simulink model "FIR_Compiler_Ex2"  (R2023a)
settings: Solver=VariableStepAuto  StartTime=0.0  StopTime=1e4  RelTol=1e-3
undefined symbols (not defined in the file): c, S, vsva2197, xcvc1902
libraries: hdlBasic x7, hdlUtilities x4, aieUtilities x4, dspsrcs4 x3, dspmlti4 x1, hdlDSPIP x1, vmcUtilities x1
settings Model: Creator=abehbood  LastModifiedBy=robg

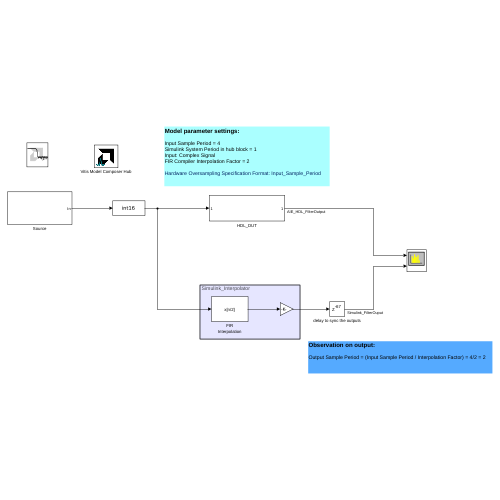
[thumbnail: Simulink's stored preview of the top-level diagram]
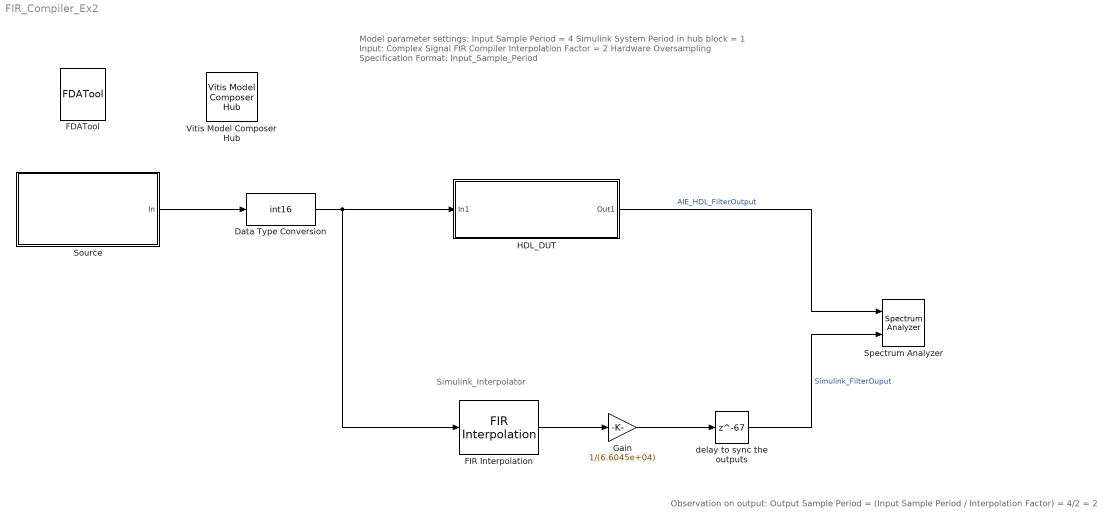
== system FIR_Compiler_Ex2 ==
  note: Simulink_Interpolator
  note: Model parameter settings:
      |
      | Input Sample Period = 4
      | Simulink System Period in hub block = 1
      | Input: Complex Signal
      | FIR Compiler Interpolation Factor = 2
      |
      | Hardware Oversampling Specification Format: Input_Sample_Period
  note: Observation on output:
      |
      | Output Sample Period = (Input Sample Period / Interpolation Factor) = 4/2 = 2
  Data Type Conversion : DataTypeConversion  OutDataTypeStr=int16  SaturateOnIntegerOverflow=off  RndMeth=Floor
  FDATool : hdlUtilities/FDATool  block_type=fdatool
      settings: infoedit=FDATool
  FIR Interpolation : dspmlti4/FIR Interpolation  FilterSource=Dialog parameters  PrivateCoeffs=0  h=[0,0,0,0,0,0,0,0,0,0,0,0,0,0,1,-1,1,-1,1,-1,1,-2,2,-2,3,-3,4,-4,5,-5,6,-7,8,-9,10,-11,12,-13,15,-17,18,-20,23,-25,27,-30,33,-36,40,-44,48,-52,56,-61,67,-72,78,-85,92,-99,107,-115,124,-134,144,-155,167,-179,192,-207,222,-238,256,-274,295,-316,340,-366,394,-424,458,-495,536,-581,633,-692,759,-837,929,-1040,1175,-1344,1564,-1862,2290,-2958,4156,-6944,20858,20858,-6944,4156,-2958,2290,-1862,1564,-1344,1175,-1040,929,-837,759,-692,633,-581,536,-495,458,-424,394,-366,340,-316,295,-274,256,-238,222,-207,192,-179,167,-155,144,-134,124,-115,107,-99,92,-85,78,-72,67,-61,56,-52,48,-44,40,-36,33,-30,27,-25,23,-20,18,-17,15,-13,12,-11,10,-9,8,-7,6,-5,5,-4,4,-3,3,-2,2,-2,1,-1,1,-1,1,-1,1,0,0,0,0,0,0,0,0,0,0,0,0,0,0]  L=2  FilterObject=FINTERP  framing=Enforce single-rate processing  outputBufInitCond=0  roundingMode=Floor  overflowMode=off  firstCoeffMode=Binary point scaling  firstCoeffWordLength=16  firstCoeffFracLength=0  firstCoeffDataTypeStr=fixdt(1,16,0)  firstCoeffMin=[]  firstCoeffMax=[]  firstCoeffLastDataTypeStr=fixdt(1,16,0)  outputDataTypeStr=Inherit: Same as accumulator  outputMin=[]  outputMax=[]  outputLastDataTypeStr=Inherit: Same as accumulator
  Gain : Gain  Gain=1/(6.6045e+04)  OutDataTypeStr=int16
  HDL_DUT : Subsystem
  Source : Subsystem
  Spectrum Analyzer : SpectrumAnalyzer  NumInputPorts=2  AveragingMethod=Exponential  ShowLegend=on  ChannelNames="[\"\"]"  DefaultConfigurationName=spbscopes.SpectrumAnalyzerBlockCfg
  Vitis Model Composer Hub : vmcUtilities/Vitis Model Composer Hub  Tag=genX  CodeGeneration=off  SubsystemName=filter_chain_DUT  StartColumn=1  NumberOfColumns=1  TargetDirectory=./code_hw_emu  exportDesign=off  analyzeDesign=off  validateDesignOnHw=off  ExportType=HW Code  IpVendor=xilinx.com  IpLibrary=hls  IpVersion=1.0  IpHWLanguage=Verilog  AieCompilerOptions={}  AieSimulatorOptions={}  CreateTestbench=off  TestbenchStackSize=10  RunRtlSim=off  RunCSim=off  RunAieSim=on  AieSimTimeout=50000  RunAieSimProfiling=off  LaunchVitisAnalyzer=off  PlotOutput=off  RunX86Sim=off  X86SimTimeout=10  GenHwImage=off  GenLibadfXo=off  GenHwValidationCode=off  PlatformType=Specify Platform  Platform=/proj/xbuilds/SWIP/2024.1_0306_2227/installs/lin64/Vitis/2024.1/base_platforms/xilinx_vck190_base_202410_1/xilinx_vck190_base_202410_1.xpfm  HwSystemType=Baremetal  HwValidationTarget=hw_emu  ProjDevice=Versal VCK190 Evaluation Platform (xcvc1902-vsva2197-2MP-e-S)  ProjDevicePart=xcvc1902-vsva2197-2MP-e-S  AIEType=AIE  SamplePeriod=-1  ClockFrequency=200  DataPathParallelism=1  xilinxfamily=versalaicore  part=xcvc1902  speed=-2MP-e-S  package=vsva2197  directory=./code_hw_emu/ip/PL/src  testbench=on  incr_netlist=off  synthesis_tool=Vivado  clock_wrapper=Clock Enables  dbl_ovrd=According to Block Masks  dcm_input_clock_period=10  sysclk_period=5  simulink_period=2  eval_field=0  IPInfoJsonString="{\"HDLSubsystem\":{\"SubsystemName\":\"PL\",\"IPName\":\"Subsystem\",\"IPLibrary\":\"VMC\",\"IPVendor\":\"User Company\",\"IPVersion\":\"1.0\",\"TargetDirectory\":\"./code_hw_emu\",\"SubsystemDir\":\"./code_hw_emu/ip/PL\"},\"SubsystemTag\":\"DUTNode\",\"AIESubsystem\":{\"SubsystemName\":\"AIE\",\"TargetDirectory\":\"./code_hw_emu\",\"SubsystemDir\":\"./code_hw_emu/ip/AIE\"}}"  LogFileName=/proj/xsjhdstaff4/abehbood/vmc_examples/gitent_ws/Examples/AIENGINE_plus_PL/AIE_HDL/multirate_filter_chain/code_hw_emu/model_composer.log  NThreads=4
  delay to sync the outputs : Delay  DelayLength=67
  wires:
  delay to sync the outputs/1 -> Spectrum Analyzer/2  "Simulink_FilterOuput"
  HDL_DUT/1(Out1) -> Spectrum Analyzer/1  "AIE_HDL_FilterOutput"
  Source/1(In) -> Data Type Conversion/1
  Gain/1 -> delay to sync the outputs/1
  Data Type Conversion/1 -> HDL_DUT/1(In1), FIR Interpolation/1
  FIR Interpolation/1 -> Gain/1

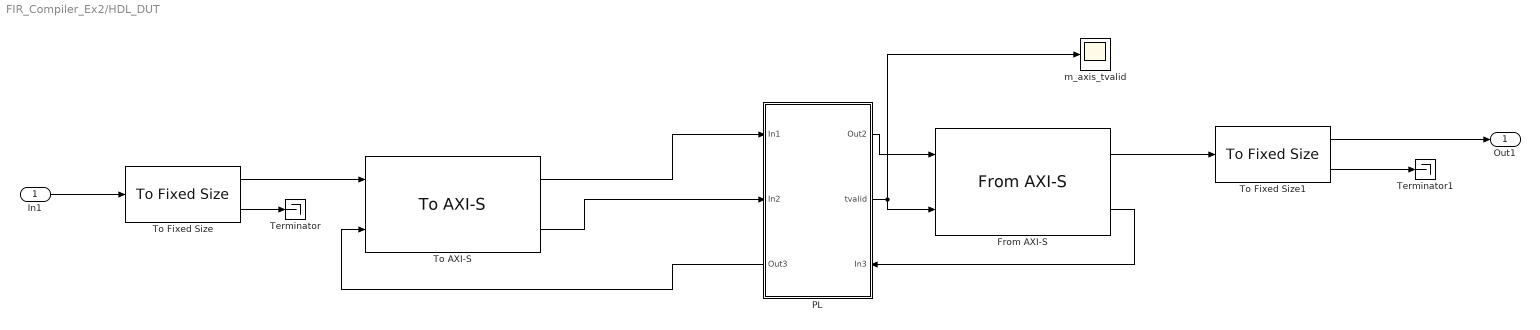
== system FIR_Compiler_Ex2/HDL_DUT ==
  In1 : Inport
  From AXI-S : aieUtilities/From AXI-S  InDataType=uint32  OutDataType=int16 (c)  OutSampleTime=OutSampleTime  SamplesPerFrame=1  RateReduceFactor=1  ManuallySpecifyOutSampleTime=off  TreadySampleTime=1
  PL : Subsystem
      settings: PortSchema="{\"entries\":[{\"content\":{\"sides\":[{\"content\":{\"connectorIds\":[\"In1\",\"In2\",\"Out3\"]},\"type\":\"ConnectorPlacement.EquallySpacedRectSide\",\"uuid\":\"b9240e68-8c33-49ba-b00e-74953cef8815\"},{\"content\":{\"connectorIds\":[\"Out1\",\"Out2\",\"In3\"],\"side\":\"RIGHT\"},\"type\":\"ConnectorPlacement.EquallySpacedRectSide\",\"uuid\":\"ae9f69ab-13df-4ed6-8e03-b2ffeca92de6\"},{\"content\":{\"side\":\"TOP\"},\"type\":\"ConnectorPlacement.EquallySpacedRectSide\",\"uuid\":\"62802255-d0c0-4e5e-87ba-02035ab73d0f\"}]},\"type\":\"ConnectorPlacement.EquallySpacedConnector\",\"uuid\":\"85ea88ef-d819-4f47-a821-adcbfe47cef7\"}],\"packageUris\":[\"http://schema.mathworks.com/mf0/Connector/R2020b\"],\"version\":\"1.0\"}"
  Terminator : Terminator
  Terminator1 : Terminator
  To AXI-S : aieUtilities/To AXI-S  OutDataType=uint32  OutSampleTime=Inherit: Same as tready
  To Fixed Size : aieUtilities/To Fixed Size  Mode=Produce a valid output signal  OutputSize=Inherit: Same as input  CopyMethod=Buffer samples to form output  HasStatusOutput=on
  To Fixed Size1 : aieUtilities/To Fixed Size  Mode=Produce a valid output signal  OutputSize=Inherit: Same as input  CopyMethod=Buffer samples to form output  HasStatusOutput=on
  m_axis_tvalid : Scope
  Out1 : Outport
  wires:
  PL/3(Out3) -> To AXI-S/2
  To AXI-S/1 -> PL/1(In1)
  To Fixed Size/1 -> To AXI-S/1
  To Fixed Size1/1 -> Out1/1
  To AXI-S/2 -> PL/2(In2)
  In1/1 -> To Fixed Size/1
  To Fixed Size/2 -> Terminator/1
  PL/1(Out2) -> From AXI-S/1
  From AXI-S/1 -> To Fixed Size1/1
  PL/2(tvalid) -> From AXI-S/2, m_axis_tvalid/1
  From AXI-S/2 -> PL/3(In3)
  To Fixed Size1/2 -> Terminator1/1

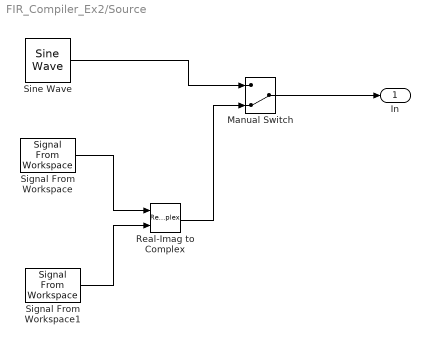
== system FIR_Compiler_Ex2/Source ==
  Manual Switch : ManualSwitch  CurrentSetting=0
  Real-Imag to Complex : RealImagToComplex
  Signal From Workspace : dspsrcs4/Signal From Workspace  X=1e3:1e5  Ts=4  nsamps=1  OutputAfterFinalValue=Cyclic repetition  ignoreOrWarnInputAndFrameLengths=off  OutputFrames=off
  Signal From Workspace1 : dspsrcs4/Signal From Workspace  X=1e3:1e5  Ts=4  nsamps=1  OutputAfterFinalValue=Cyclic repetition  ignoreOrWarnInputAndFrameLengths=off  OutputFrames=off
  Sine Wave : dspsrcs4/Sine Wave  Amplitude=2^10  Frequency=1e-6  Phase=0  SampleMode=Discrete  OutComplex=Complex  CompMethod=Trigonometric fcn  TableSize=Speed  SampleTime=4  SamplesPerFrame=1  ResetState=Restart at time zero  OutputFrames=off  dataType=double  wordLen=16  udDataType=sfix(16)  fracBitsMode=Best precision  numFracBits=15  OutDataTypeStr=double  LastOutDataTypeStr=double
  In : Outport
  wires:
  Signal From Workspace/1 -> Real-Imag to Complex/1
  Real-Imag to Complex/1 -> Manual Switch/2
  Sine Wave/1 -> Manual Switch/1
  Signal From Workspace1/1 -> Real-Imag to Complex/2
  Manual Switch/1 -> In/1

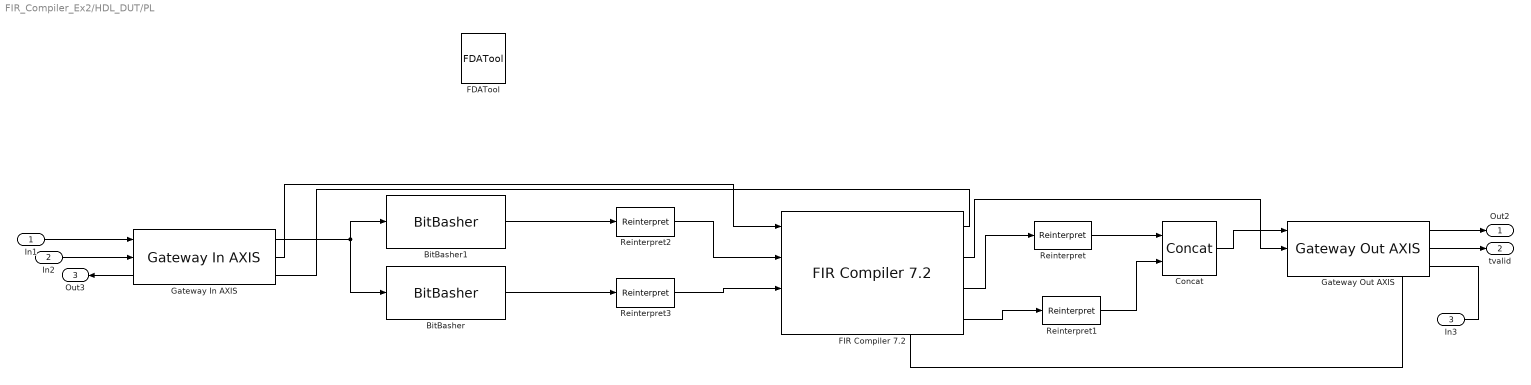
== system FIR_Compiler_Ex2/HDL_DUT/PL ==
  In1 : Inport
  In2 : Inport  Port=2
  In3 : Inport  Port=3
  BitBasher : hdlBasic/BitBasher  bitexpr=real={in[15:0]}  display_expr=on  sr_1=real  arith_type1=Unsigned  bin_pt1=0  sr_2=2  arith_type2=Unsigned  bin_pt2=0  sr_3=3  arith_type3=Unsigned  bin_pt3=0  sr_4=4  arith_type4=Unsigned  bin_pt4=0  XmcBlockStatus=1  maskContainerNames=group1  block_type=bitbasher  block_config=sysgen:BitBasher_config
  BitBasher1 : hdlBasic/BitBasher  bitexpr=imag={in[31:16]}  display_expr=on  sr_1=imag  arith_type1=Unsigned  bin_pt1=0  sr_2=2  arith_type2=Unsigned  bin_pt2=0  sr_3=3  arith_type3=Unsigned  bin_pt3=0  sr_4=4  arith_type4=Unsigned  bin_pt4=0  XmcBlockStatus=1  maskContainerNames=group1  block_type=bitbasher  block_config=sysgen:BitBasher_config
  Concat : hdlBasic/Concat  num_inputs=2  XmcBlockStatus=1  maskContainerNames=group1  block_type=concat  block_config=sysgen:Concat_config
  FDATool : hdlUtilities/FDATool  block_type=fdatool
      settings: infoedit=FDATool
  FIR Compiler 7.2 : hdlDSPIP/FIR Compiler 7.2   coefficientvector=[0,0,0,0,0,0,0,0,0,0,0,0,0,0,1,-1,1,-1,1,-1,1,-2,2,-2,3,-3,4,-4,5,-5,6,-7,8,-9,10,-11,12,-13,15,-17,18,-20,23,-25,27,-30,33,-36,40,-44,48,-52,56,-61,67,-72,78,-85,92,-99,107,-115,124,-134,144,-155,167,-179,192,-207,222,-238,256,-274,295,-316,340,-366,394,-424,458,-495,536,-581,633,-692,759,-837,929,-1040,1175,-1344,1564,-1862,2290,-2958,4156,-6944,20858,20858,-6944,4156,-2958,2290,-1862,1564,-1344,1175,-1040,929,-837,759,-692,633,-581,536,-495,458,-424,394,-366,340,-316,295,-274,256,-238,222,-207,192,-179,167,-155,144,-134,124,-115,107,-99,92,-85,78,-72,67,-61,56,-52,48,-44,40,-36,33,-30,27,-25,23,-20,18,-17,15,-13,12,-11,10,-9,8,-7,6,-5,5,-4,4,-3,3,-2,2,-2,1,-1,1,-1,1,-1,1,0,0,0,0,0,0,0,0,0,0,0,0,0,0]  coefficient_sets=1  coefficient_reload=off  filter_type=Interpolation  rate_change_type=Integer  interpolation_rate=2  decimation_rate=1  zero_pack_factor=1  channel_sequence=Basic  number_channels=1  pattern_list='P4-0,P4-1,P4-2,P4-3,P4-4'  number_paths=2  ratespecification=Input_Sample_Period  sampleperiod=2  hardwareoversamplingrate=1  coefficient_sign=Signed  quantization=Integer_Coefficients  coefficient_width=16  bestprecision=off  coefficient_fractional_bits=0  coefficient_structure=Inferred  output_rounding_mode=Truncate_LSBs  output_width=16  filter_architecture=Systolic_Multiply_Accumulate  optimization_goal=Area  optimization_list='None'  data_buffer_type=Automatic  coefficient_buffer_type=Automatic  input_buffer_type=Automatic  output_buffer_type=Automatic  preference_for_other_storage=Automatic  multi_column_support=Automatic  columnconfig='50'  inter_column_pipe_length=4  data_has_tlast=Not_Required  m_data_has_tready=on  s_data_has_fifo=on  s_data_has_tuser=Not_Required  m_data_has_tuser=Not_Required  s_config_sync_mode=On_Vector  s_config_method=Single  num_reload_slots=1  has_aclken=off  has_aresetn=off  reset_data_vector=on  trim_axipin_name=on  simulation_type=hybrid_sim  simulation_model=sysgen:xfirv7_2_cmodel  data_path_portlist={ 's_axis_data_tdata', 'm_axis_data_tdata' }  passband_min=0.0  passband_max=0.5  stopband_min=0.5  stopband_max=1.0  filter_selection=1  gui_behaviour='Sysgen_GUI'  data_sign=Signed  data_width=16  data_fractional_bits=0  data_tuser_width=1  wrapper_available=true  ip_wrap_arbitrary_binary_point=true  ip_name=FIR Compiler  ip_version=7.2  dsptool_ready=true  ipcore_usecache=true  ipcore_useipmodelcache=true  port_translation_map={ 'aclken' => 'en', 'aresetn' => 'rst' }  run_core_at_system_period=true  ipcore_xco_need_fpga_part=true  ipcore_fpga_part=[]  XmcBlockStatus=1  maskContainerNames=tabcontainer1  block_type=fir_compiler_v7_2  block_config=sysgen:rodinimport_config  block_width=820  block_height=600
  Gateway In AXIS : hdlUtilities/Gateway In AXIS  gui_display_data_type=Fixed-point  arith_type=Unsigned  n_bits=32  bin_pt=0  preci_type=Custom  exp_width=16  frac_width=24  quantization=Truncate  overflow=Flag as error  OutSampleTime=4  block_type=gatewayinaxi  XmcBlockStatus=1
  Gateway Out AXIS : hdlUtilities/Gateway Out AXIS  mask_sample_period=2  block_type=gatewayoutaxi
  Reinterpret : hdlBasic/Reinterpret  force_arith_type=on  arith_type=Unsigned  force_bin_pt=off  bin_pt=0  XmcBlockStatus=1  maskContainerNames=group1  block_type=reinterpret  block_config=sysgen:Reinterpret_config
  Reinterpret1 : hdlBasic/Reinterpret  force_arith_type=on  arith_type=Unsigned  force_bin_pt=off  bin_pt=0  XmcBlockStatus=1  maskContainerNames=group1  block_type=reinterpret  block_config=sysgen:Reinterpret_config
  Reinterpret2 : hdlBasic/Reinterpret  force_arith_type=on  arith_type="Signed  (2's comp)"  force_bin_pt=off  bin_pt=0  XmcBlockStatus=1  maskContainerNames=group1  block_type=reinterpret  block_config=sysgen:Reinterpret_config
  Reinterpret3 : hdlBasic/Reinterpret  force_arith_type=on  arith_type="Signed  (2's comp)"  force_bin_pt=off  bin_pt=0  XmcBlockStatus=1  maskContainerNames=group1  block_type=reinterpret  block_config=sysgen:Reinterpret_config
  Out2 : Outport
  tvalid : Outport  Port=2
  Out3 : Outport  Port=3
  wires:
  In1/1 -> Gateway In AXIS/1
  BitBasher/1 -> Reinterpret3/1
  BitBasher1/1 -> Reinterpret2/1
  FIR Compiler 7.2/3 -> Reinterpret/1
  FIR Compiler 7.2/4 -> Reinterpret1/1
  Reinterpret1/1 -> Concat/2
  Reinterpret3/1 -> FIR Compiler 7.2/3
  Reinterpret/1 -> Concat/1
  Gateway In AXIS/1 -> BitBasher/1, BitBasher1/1
  Reinterpret2/1 -> FIR Compiler 7.2/2
  Gateway In AXIS/2 -> FIR Compiler 7.2/1
  In2/1 -> Gateway In AXIS/2
  FIR Compiler 7.2/1 -> Gateway In AXIS/3
  Gateway In AXIS/3 -> Out3/1
  Gateway Out AXIS/1 -> Out2/1
  FIR Compiler 7.2/2 -> Gateway Out AXIS/2
  Concat/1 -> Gateway Out AXIS/1
  Gateway Out AXIS/2 -> tvalid/1
  In3/1 -> Gateway Out AXIS/3
  Gateway Out AXIS/3 -> FIR Compiler 7.2/4
